simulink model "Aufgabe_10_2_6_Vereinzeler_2"  (R2023a)
settings: Solver=ode3  StartTime=0.0  StopTime=10.0  FixedStep=0.01  RelTol=1e-3  EnableMultiTasking=on
undefined symbols (not defined in the file): sigbuilder_block
libraries: simulink x7
settings Model: Creator=Junle  LastModifiedBy=ASUS
settings RTWCC: GPUComputeCapability=5.0

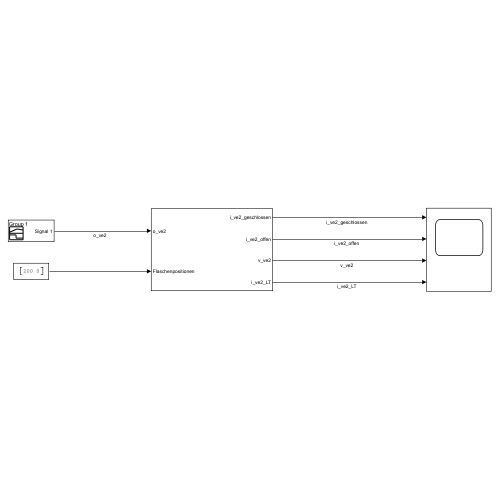
[thumbnail: Simulink's stored preview of the top-level diagram]
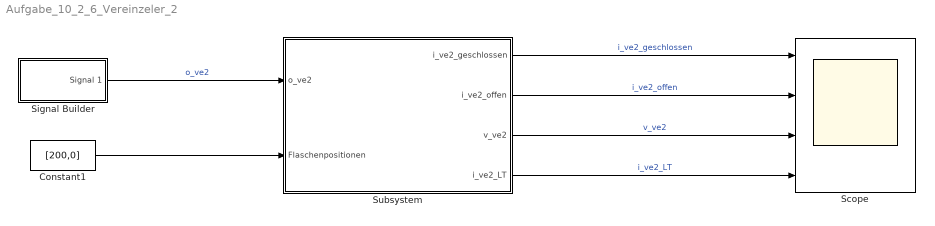
== system Aufgabe_10_2_6_Vereinzeler_2 ==
  Constant1 : Constant  Value=[200,0]
  Scope : Scope  NumInputPorts=4
  Signal Builder : Subsystem  Tag=STV Subsys  LoadFcn=sigbuilder_block('load');  StartFcn=sigbuilder_block('start');  StopFcn=sigbuilder_block('stop');  ClipboardFcn=sigbuilder_block('clipboard');  mask(Sigbuilder block){tuvar=[0:10]}
      mask help: Simulink:masks:SigbuilderBlock_MD
      mask init:
      | if ~strcmp(get_param(bdroot(gcbh),'SimulationStatus'),'stopped') tuvar = sigbuilder_block('maskInit'); end
      settings: CopyFcn=sigbuilder_block('copy');  DeleteFcn=sigbuilder_block('delete');  ModelCloseFcn=sigbuilder_block('modelClose');  PreSaveFcn=sigbuilder_block('preSave');  PauseFcn=sigbuilder_block('pause');  ContinueFcn=sigbuilder_block('continue');  NameChangeFcn=sigbuilder_block('namechange');  OpenFcn=sigbuilder_block('open',[247.2 153.6 544.2 355.2 ]);  CloseFcn=sigbuilder_block('close');
      mask Display: plot(0, 0, 100, 100,[2, 2, 32, 32, 2], [68, 8, 8, 68, 68],[32, 2], [38, 38], [32, 19, 2],[53, 60, 44], [32, 17, 17, 2],[16, 16, 31, 31]);txt = getActiveGroup(gcbh);text(2, 100, txt,'verticalAlignment', 'top');
  Subsystem : Subsystem
  wires:
  Constant1/1 -> Subsystem/2(Flaschenpositionen)
  Signal Builder/1(Signal 1) -> Subsystem/1(o_ve2)  "o_ve2"
  Subsystem/1(i_ve2_geschlossen) -> Scope/1  "i_ve2_geschlossen"
  Subsystem/2(i_ve2_offen) -> Scope/2  "i_ve2_offen"
  Subsystem/3(v_ve2) -> Scope/3  "v_ve2"
  Subsystem/4(i_ve2_LT) -> Scope/4  "i_ve2_LT"

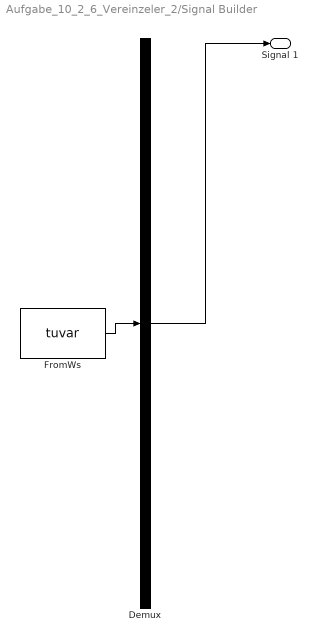
== system Aufgabe_10_2_6_Vereinzeler_2/Signal Builder ==
  Demux : Demux  Tag=STV Demux  Outputs=1
      settings: DisplayOption=none
  FromWs : FromWorkspace  Tag=STV FromWs  VariableName=tuvar
      SigBuilderData=|
      | common.afterFinalStr = 'Extrapolate'
      | common.sampleTime = 0
      | dataSet.timeRange = [0 10]
      | dataSet.name = 'Group 1'
      | sbobj.Groups.Name = 'Group 1'
      | sbobj.Groups.Signals.Name = 'Signal 1'
      | sbobj.Groups.Signals.XData = [0 1 1 3 3 6 6 8 8 10]
      | sbobj.Groups.Signals.YData = [0 0 1 1 0 0 1 1 0 0]
  Signal 1 : Outport  Tag=STV Outport
  wires:
  Demux/1 -> Signal 1/1
  FromWs/1 -> Demux/1

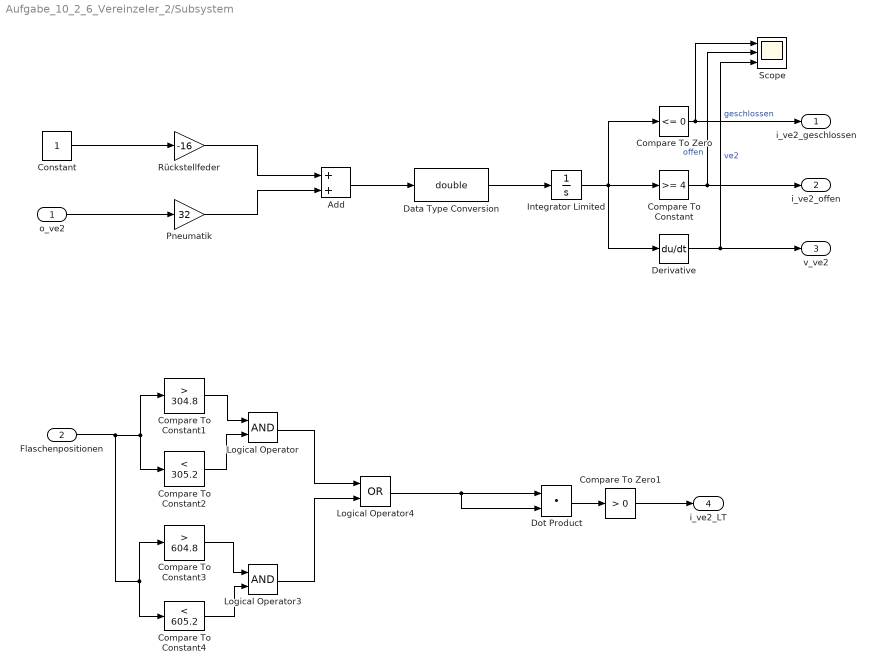
== system Aufgabe_10_2_6_Vereinzeler_2/Subsystem ==
  o_ve2 : Inport
  Flaschenpositionen : Inport  Port=2
  Add : Sum
  Compare To Constant : simulink/Logic and Bit Operations/Compare To Constant  relop=>=  const=4  OutDataTypeStr=boolean
  Compare To Constant1 : simulink/Logic and Bit Operations/Compare To Constant  relop=>  const=304.8  OutDataTypeStr=boolean
  Compare To Constant2 : simulink/Logic and Bit Operations/Compare To Constant  relop=<  const=305.2  OutDataTypeStr=boolean
  Compare To Constant3 : simulink/Logic and Bit Operations/Compare To Constant  relop=>  const=604.8  OutDataTypeStr=boolean
  Compare To Constant4 : simulink/Logic and Bit Operations/Compare To Constant  relop=<  const=605.2  OutDataTypeStr=boolean
  Compare To Zero : simulink/Logic and Bit Operations/Compare To Zero  relop=<=  OutDataTypeStr=boolean
  Compare To Zero1 : simulink/Logic and Bit Operations/Compare To Zero  relop=>  OutDataTypeStr=boolean
  Constant : Constant
  Data Type Conversion : DataTypeConversion  OutDataTypeStr=double  SaturateOnIntegerOverflow=off  RndMeth=Floor
  Derivative : Derivative
  Dot Product : DotProduct  OutDataTypeStr=Inherit: Inherit via internal rule
  Integrator Limited : Integrator  LimitOutput=on  UpperSaturationLimit=4  LowerSaturationLimit=0
  Logical Operator : Logic  AllPortsSameDT=off  OutDataTypeStr=boolean
  Logical Operator3 : Logic  AllPortsSameDT=off  OutDataTypeStr=boolean
  Logical Operator4 : Logic  Operator=OR  AllPortsSameDT=off  OutDataTypeStr=boolean
  Pneumatik : Gain  Gain=32
  Rückstellfeder : Gain  Gain=-16
  Scope : Scope  NumInputPorts=3
  i_ve2_geschlossen : Outport
  i_ve2_offen : Outport  Port=2
  v_ve2 : Outport  Port=3
  i_ve2_LT : Outport  Port=4  VectorParamsAs1DForOutWhenUnconnected=off
  wires:
  Constant/1 -> Rückstellfeder/1
  o_ve2/1 -> Pneumatik/1
  Integrator Limited/1 -> Compare To Constant/1, Derivative/1, Compare To Zero/1
  Data Type Conversion/1 -> Integrator Limited/1
  Rückstellfeder/1 -> Add/1
  Compare To Constant/1 -> Scope/2, i_ve2_offen/1  "offen"
  Compare To Zero/1 -> Scope/1, i_ve2_geschlossen/1  "geschlossen"
  Pneumatik/1 -> Add/2
  Add/1 -> Data Type Conversion/1
  Derivative/1 -> Scope/3, v_ve2/1  "ve2"
  Logical Operator4/1 -> Dot Product/2, Dot Product/1
  Compare To Constant4/1 -> Logical Operator3/2
  Compare To Constant3/1 -> Logical Operator3/1
  Logical Operator3/1 -> Logical Operator4/2
  Logical Operator/1 -> Logical Operator4/1
  Flaschenpositionen/1 -> Compare To Constant4/1, Compare To Constant3/1, Compare To Constant1/1, Compare To Constant2/1
  Compare To Zero1/1 -> i_ve2_LT/1
  Compare To Constant2/1 -> Logical Operator/2
  Dot Product/1 -> Compare To Zero1/1
  Compare To Constant1/1 -> Logical Operator/1
